simulink model "sampleModel2040"  (R2023a)
settings: Solver=VariableStepAuto  StartTime=0.0  StopTime=10.0  RelTol=1e-3
libraries: hdlsllib x1
settings Model: Creator=user1  LastModifiedBy=user1

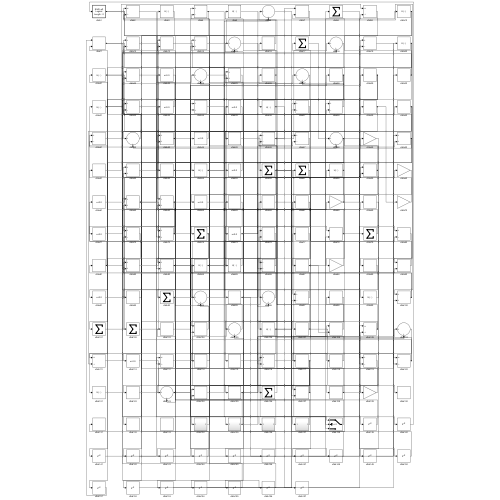
[thumbnail: Simulink's stored preview of the top-level diagram]
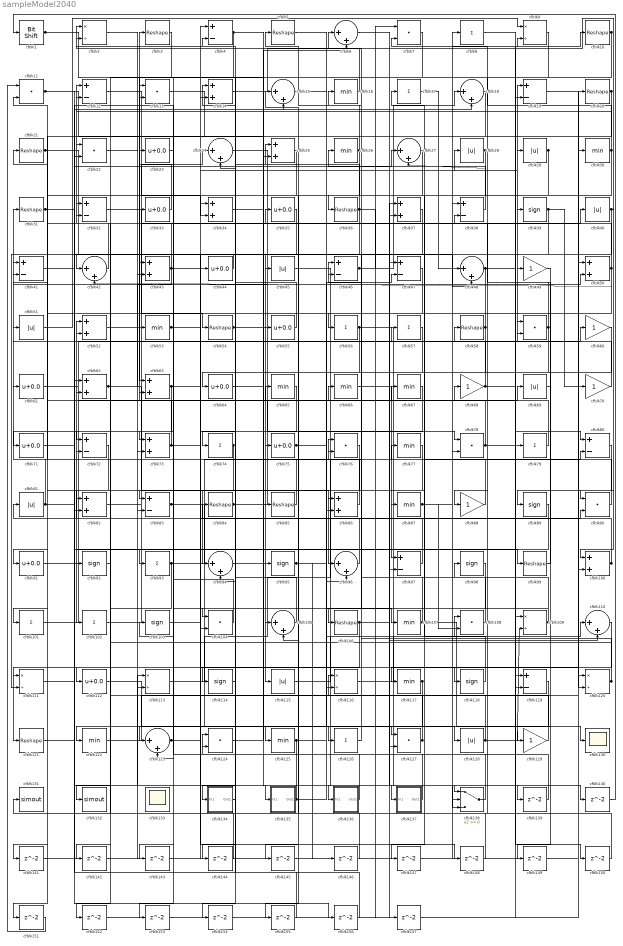
== system sampleModel2040 ==
  cfblk1 : hdlsllib/Logic and Bit Operations/Bit Shift  mode=Shift Left Logical  N=0
  cfblk{3,5,10,20..21,31,36,54,58,84..85,99,106,121} (14 alike) : Reshape
  cfblk{14,25,34,37,43,50,52,62..63,73,82,86,100} (13 alike) : Sum
  cfblk{8,17,56..57,74,79,93,101..102,126} (10 alike) : Sum  Inputs=+
  cfblk{39,89,92,95,98,103,114,118} (8 alike) : Signum
  cfblk{7,11,13,22,59,76,78,90,104,108,124,127} (12 alike) : DotProduct  OutDataTypeStr=Inherit: Inherit via internal rule
  cfblk{6,15,18,24,27,42,48,94,96,105,110,123} (12 alike) : Sum  Inputs=|++
  cfblk{16,26,30,53,65..67,77,87,107,117,122,125} (13 alike) : MinMax
  cfblk{2,9,109,111,113,116,120} (7 alike) : Product  Inputs=*/  RndMeth=Zero  SaturateOnIntegerOverflow=on
  cfblk{23,33,35,44,55,61,64,71,75,91,112} (11 alike) : Bias  Bias=0.0  SaturateOnIntegerOverflow=off
  cfblk{28..29,40,45,51,69,81,115,128} (9 alike) : Abs  SaturateOnIntegerOverflow=off
  cfblk{4,12,19,32,38,41,46..47,72,80,83,97,119} (13 alike) : Sum  Inputs=+-
  cfblk{49,60,68,70,88,129} (6 alike) : Gain
  cfblk130 : Scope
  cfblk131 : ToWorkspace  VariableName=simout  SaveFormat=Timeseries  SampleTime=-1
  cfblk132 : ToWorkspace  VariableName=simout  SaveFormat=Timeseries  SampleTime=-1
  cfblk133 : Scope
      settings: Floating=on
  cfblk134 : Subsystem
      settings: LibrarySourceBlock=|
      | hdlsllib/Ports &
      | Subsystems/Subsystem
  cfblk135 : Subsystem
      settings: LibrarySourceBlock=|
      | hdlsllib/Ports &
      | Subsystems/Subsystem
  cfblk136 : Subsystem
      settings: LibrarySourceBlock=|
      | hdlsllib/Ports &
      | Subsystems/Subsystem
  cfblk137 : Subsystem
      settings: LibrarySourceBlock=|
      | hdlsllib/Ports &
      | Subsystems/Subsystem
  cfblk138 : Switch  SaturateOnIntegerOverflow=off  InputSameDT=off
  cfblk{139..157} (19 alike) : Delay  SampleTime=1
  wires:
  cfblk24/1 -> cfblk78/1
  cfblk45/1 -> cfblk137/1(In1)
  cfblk37/1 -> cfblk115/1
  cfblk97/1 -> cfblk52/1
  cfblk39/1 -> cfblk70/1, cfblk104/2
  cfblk73/1 -> cfblk3/1, cfblk138/3, cfblk72/1
  cfblk93/1 -> cfblk76/1, cfblk132/1
  cfblk51/1 -> cfblk9/1
  cfblk82/1 -> cfblk65/1
  cfblk10/1 -> cfblk131/1, cfblk83/1
  cfblk60/1 -> cfblk88/1
  cfblk43/1 -> cfblk12/1, cfblk41/2, cfblk75/1
  cfblk56/1 -> cfblk138/1, cfblk38/2, cfblk114/1, cfblk110/2
  cfblk96/1 -> cfblk81/1
  cfblk95/1 -> cfblk59/2, cfblk146/1
  cfblk17/1 -> cfblk48/1
  cfblk44/1 -> cfblk42/1
  cfblk14/1 -> cfblk100/1
  cfblk4/1 -> cfblk112/1, cfblk86/2
  cfblk102/1 -> cfblk40/1
  cfblk120/1 -> cfblk16/1, cfblk62/2
  cfblk46/1 -> cfblk18/1, cfblk7/1
  cfblk21/1 -> cfblk45/1, cfblk96/2
  cfblk40/1 -> cfblk106/1, cfblk111/2, cfblk90/1
  cfblk9/1 -> cfblk63/1
  cfblk59/1 -> cfblk33/1, cfblk147/1
  cfblk75/1 -> cfblk68/1, cfblk60/1
  cfblk111/1 -> cfblk18/2
  cfblk87/1 -> cfblk9/2, cfblk108/2
  cfblk107/1 -> cfblk130/1, cfblk63/2
  cfblk91/1 -> cfblk66/1
  cfblk15/1 -> cfblk107/1
  cfblk117/1 -> cfblk152/1, cfblk153/1, cfblk154/1
  cfblk115/1 -> cfblk79/1
  cfblk66/1 -> cfblk97/1
  cfblk32/1 -> cfblk54/1
  cfblk127/1 -> cfblk103/1, cfblk72/2
  cfblk52/1 -> cfblk24/1
  cfblk29/1 -> cfblk125/1, cfblk93/1, cfblk119/2
  cfblk1/1 -> cfblk55/1, cfblk53/1
  cfblk116/1 -> cfblk8/1
  cfblk42/1 -> cfblk22/1
  cfblk19/1 -> cfblk120/1
  cfblk124/1 -> cfblk77/1
  cfblk12/1 -> cfblk34/2
  cfblk83/1 -> cfblk126/1, cfblk90/2
  cfblk125/1 -> cfblk124/1, cfblk110/1, cfblk108/1
  cfblk26/1 -> cfblk5/1, cfblk111/1
  cfblk76/1 -> cfblk94/1
  cfblk101/1 -> cfblk19/1
  cfblk28/1 -> cfblk87/1, cfblk43/2, cfblk27/2
  cfblk41/1 -> cfblk27/1
  cfblk128/1 -> cfblk109/2, cfblk46/2
  cfblk104/1 -> cfblk13/1
  cfblk123/1 -> cfblk69/1, cfblk148/1
  cfblk81/1 -> cfblk31/1, cfblk15/2
  cfblk16/1 -> cfblk6/1
  cfblk105/1 -> cfblk14/1
  cfblk122/1 -> cfblk20/1
  cfblk53/1 -> cfblk28/1, cfblk120/2
  cfblk13/1 -> cfblk95/1
  cfblk61/1 -> cfblk44/1
  cfblk72/1 -> cfblk102/1
  cfblk106/1 -> cfblk121/1, cfblk118/1, cfblk59/1
  cfblk54/1 -> cfblk136/1(In1), cfblk6/2
  cfblk38/1 -> cfblk26/1
  cfblk92/1 -> cfblk32/1
  cfblk99/1 -> cfblk49/1
  cfblk58/1 -> cfblk56/1, cfblk127/2
  cfblk57/1 -> cfblk104/1
  cfblk78/1 -> cfblk80/1, cfblk46/1
  cfblk112/1 -> cfblk128/1
  cfblk88/1 -> cfblk17/1
  cfblk129/1 -> cfblk116/1
  cfblk8/1 -> cfblk119/1
  cfblk77/1 -> cfblk116/2
  cfblk138/1 -> cfblk82/1
  cfblk86/1 -> cfblk61/1
  cfblk3/1 -> cfblk122/1
  cfblk85/1 -> cfblk41/1
  cfblk63/1 -> cfblk135/1(In1), cfblk141/1
  cfblk100/1 -> cfblk35/1, cfblk15/1
  cfblk49/1 -> cfblk129/1
  cfblk62/1 -> cfblk50/2, cfblk96/1
  cfblk5/1 -> cfblk127/1
  cfblk20/1 -> cfblk134/1(In1), cfblk151/1
  cfblk113/1 -> cfblk37/2
  cfblk47/1 -> cfblk91/1
  cfblk70/1 -> cfblk43/1
  cfblk68/1 -> cfblk32/2, cfblk10/1
  cfblk31/1 -> cfblk13/2, cfblk156/1
  cfblk50/1 -> cfblk92/1, cfblk11/2, cfblk42/2, cfblk86/1
  cfblk33/1 -> cfblk23/1
  cfblk35/1 -> cfblk74/1
  cfblk118/1 -> cfblk67/1
  cfblk98/1 -> cfblk123/1
  cfblk103/1 -> cfblk29/1
  cfblk109/1 -> cfblk105/1, cfblk98/1
  cfblk48/1 -> cfblk82/2, cfblk73/1, cfblk150/1
  cfblk135/1(Out1) -> cfblk47/2, cfblk124/2
  cfblk7/1 -> cfblk64/1
  cfblk74/1 -> cfblk101/1, cfblk83/2
  cfblk23/1 -> cfblk123/2
  cfblk94/1 -> cfblk80/2
  cfblk121/1 -> cfblk138/2
  cfblk90/1 -> cfblk57/1
  cfblk114/1 -> cfblk94/2
  cfblk11/1 -> cfblk113/2, cfblk48/2
  cfblk25/1 -> cfblk71/1
  cfblk136/1(Out1) -> cfblk25/1
  cfblk64/1 -> cfblk39/1
  cfblk137/1(Out1) -> cfblk51/1
  cfblk126/1 -> cfblk76/2
  cfblk79/1 -> cfblk21/1
  cfblk34/1 -> cfblk99/1
  cfblk108/1 -> cfblk2/1
  cfblk134/1(Out1) -> cfblk84/1
  cfblk84/1 -> cfblk38/1, cfblk58/1
  cfblk65/1 -> cfblk85/1
  cfblk80/1 -> cfblk89/1
  cfblk30/1 -> cfblk36/1, cfblk12/2, cfblk7/2
  cfblk36/1 -> cfblk73/2, cfblk2/2, cfblk157/1
  cfblk110/1 -> cfblk117/1
  cfblk55/1 -> cfblk4/2
  cfblk71/1 -> cfblk22/2
  cfblk2/1 -> cfblk25/2
  cfblk6/1 -> cfblk139/1
  cfblk139/1 -> cfblk4/1
  cfblk22/1 -> cfblk140/1
  cfblk140/1 -> cfblk1/1
  cfblk141/1 -> cfblk14/2
  cfblk89/1 -> cfblk142/1
  cfblk142/1 -> cfblk113/1
  cfblk18/1 -> cfblk143/1
  cfblk143/1 -> cfblk100/2
  cfblk119/1 -> cfblk144/1
  cfblk144/1 -> cfblk34/1
  cfblk27/1 -> cfblk145/1
  cfblk145/1 -> cfblk78/2
  cfblk146/1 -> cfblk52/2
  cfblk147/1 -> cfblk109/1
  cfblk148/1 -> cfblk37/1
  cfblk69/1 -> cfblk149/1
  cfblk149/1 -> cfblk50/1
  cfblk150/1 -> cfblk105/2
  cfblk151/1 -> cfblk11/1
  cfblk152/1 -> cfblk47/1
  cfblk153/1 -> cfblk19/2
  cfblk154/1 -> cfblk97/2
  cfblk67/1 -> cfblk155/1
  cfblk155/1 -> cfblk24/2
  cfblk156/1 -> cfblk62/1
  cfblk157/1 -> cfblk30/1

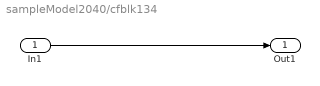
== system sampleModel2040/cfblk134 ==
  In1 : Inport
  Out1 : Outport
  wires:
  In1/1 -> Out1/1

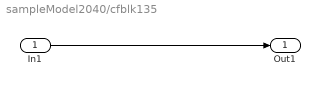
== system sampleModel2040/cfblk135 ==
  In1 : Inport
  Out1 : Outport
  wires:
  In1/1 -> Out1/1

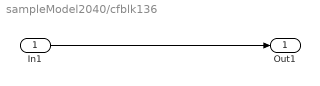
== system sampleModel2040/cfblk136 ==
  In1 : Inport
  Out1 : Outport
  wires:
  In1/1 -> Out1/1

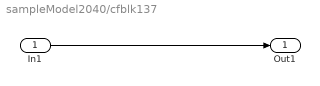
== system sampleModel2040/cfblk137 ==
  In1 : Inport
  Out1 : Outport
  wires:
  In1/1 -> Out1/1
